simulink model "flightSimulation"  (R2018a)
settings: Solver=FixedStepAuto  StartTime=0  StopTime=end_time  FixedStep=0.005  RelTol=1e-3  EnableMultiTasking=on
values from neighbouring files (symbols this model uses):
  initPosLLA = [37.6287386167 -122.393391133 100]    [cmdh.mat]    (also in cmdyaw.mat)
  mass = 1.53    [cmdh.mat]    (also in cmdyaw.mat)
  Ts = 0.01    [cmdh.mat]    (also in cmdyaw.mat)
undefined symbols (not defined in the file or in its folder): B, Earth, ft, m, p_limits, s, sigbuilder_block, sw_turb, umax, umin, Vehicle, WGS84
libraries: simulink x23, aerolibactuator x15, dspswit3 x12, dspsrcs4 x10, dsparch4 x7, aerolibconvert2 x4, aerolibanimutils x2, qcatlib x2, aerolibfltsims x2, aerolibutil x2, shared6dof x1, aerolibtransform2 x1
(part 2 of 4)

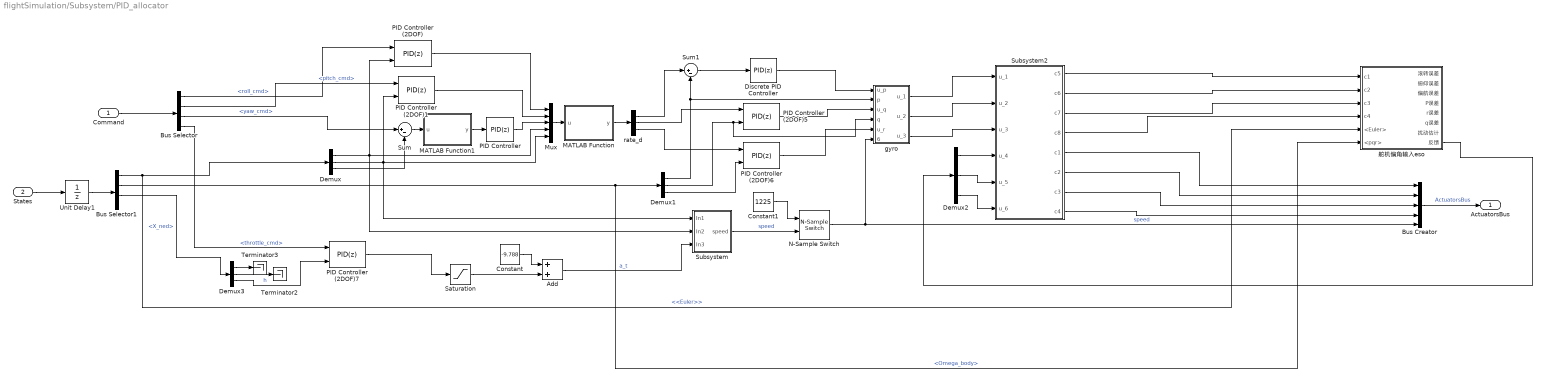
== system flightSimulation/Subsystem/PID_allocator ==
  Command : Inport
  States : Inport  Port=2  OutDataTypeStr=Bus: StatesBus
  Add : Sum
  Bus Creator : BusCreator  Inputs=5  OutDataTypeStr=Bus: ActuatorsBus
  Bus Selector : BusSelector  OutputSignals=roll_cmd,pitch_cmd,yaw_cmd,throttle_cmd
  Bus Selector1 : BusSelector  OutputSignals=<Euler>,Omega_body,X_ned,V_ned
  Constant : Constant  Value=-9.788
  Constant1 : Constant  Value=1225
  Demux{,1..3} (4 alike) : Demux  Outputs=3
  Discrete PID Controller : simulink/Continuous/PID Controller  Controller=PID  TimeDomain=Discrete-time  SampleTime=-1  IntegratorMethod=Forward Euler  FilterMethod=Forward Euler  Form=Parallel  UseFilter=on  ControllerParametersSource=internal  P=0.4  I=0.32  D=0  N=100  InitialConditionSource=internal  InitialConditionForIntegrator=0  InitialConditionForFilter=0  ExternalReset=none  LimitOutput=off  UpperSaturationLimit=inf  LowerSaturationLimit=-inf  LinearizeAsGain=off  AntiWindupMode=none  Kb=1  TrackingMode=off  Kt=1  PParamMin=[]  PParamMax=[]  IParamMin=[]  IParamMax=[]  DParamMin=[]  DParamMax=[]  NParamMin=[]  NParamMax=[]  KbParamMin=[]  KbParamMax=[]  KtParamMin=[]  KtParamMax=[]  POutMin=[]  POutMax=[]  IOutMin=[]  IOutMax=[]  DOutMin=[]  DOutMax=[]  NOutMin=[]  NOutMax=[]  KbOutMin=[]  KbOutMax=[]  KtOutMin=[]  KtOutMax=[]  IntegratorOutMin=[]  IntegratorOutMax=[]  FilterOutMin=[]  FilterOutMax=[]  SumOutMin=[]  SumOutMax=[]  SumI1OutMin=[]  SumI1OutMax=[]  SumI2OutMin=[]  SumI2OutMax=[]  SumI3OutMin=[]  SumI3OutMax=[]  SumDOutMin=[]  SumDOutMax=[]  SaturationOutMin=[]  SaturationOutMax=[]  IntegratorContinuousStateAttributes=''  IntegratorStateMustResolveToSignalObject=off  IntegratorRTWStateStorageClass=Auto  FilterContinuousStateAttributes=''  FilterStateMustResolveToSignalObject=off  FilterRTWStateStorageClass=Auto  DifferentiatorICPrevScaledInput=0  DifferentiatorOutMin=[]  DifferentiatorOutMax=[]  FilterDiffOutCoefMin=[]  FilterDiffOutCoefMax=[]  SumDenOutMin=[]  SumDenOutMax=[]  SumNumOutMin=[]  SumNumOutMax=[]  ReciprocalOutMin=[]  ReciprocalOutMax=[]  DivideOutMin=[]  DivideOutMax=[]  TunerSelectOption=Transfer Function Based (PID Tuner App)
  MATLAB Function : MATLAB Function  TreatAsAtomicUnit=on
  MATLAB Function1 : MATLAB Function  TreatAsAtomicUnit=on
  Mux : Mux  Inputs=5
  N-Sample Switch : dspswit3/N-Sample Switch  N=3  reset=off  TriggerType=Rising edge  Ts=0.01
      settings: SourceProductName=DSP System Toolbox  SourceProductBaseCode=DS
  PID Controller : simulink/Continuous/PID Controller  Controller=PID  TimeDomain=Discrete-time  SampleTime=-1  IntegratorMethod=Forward Euler  FilterMethod=Forward Euler  Form=Parallel  UseFilter=on  ControllerParametersSource=internal  P=3  I=0.2  D=0  N=100  InitialConditionSource=internal  InitialConditionForIntegrator=0  InitialConditionForFilter=0  ExternalReset=none  LimitOutput=off  UpperSaturationLimit=1*pi  LowerSaturationLimit=-1*pi  LinearizeAsGain=on  AntiWindupMode=none  Kb=1  TrackingMode=off  Kt=1  PParamMin=[]  PParamMax=[]  IParamMin=[]  IParamMax=[]  DParamMin=[]  DParamMax=[]  NParamMin=[]  NParamMax=[]  KbParamMin=[]  KbParamMax=[]  KtParamMin=[]  KtParamMax=[]  POutMin=[]  POutMax=[]  IOutMin=[]  IOutMax=[]  DOutMin=[]  DOutMax=[]  NOutMin=[]  NOutMax=[]  KbOutMin=[]  KbOutMax=[]  KtOutMin=[]  KtOutMax=[]  IntegratorOutMin=[]  IntegratorOutMax=[]  FilterOutMin=[]  FilterOutMax=[]  SumOutMin=[]  SumOutMax=[]  SumI1OutMin=[]  SumI1OutMax=[]  SumI2OutMin=[]  SumI2OutMax=[]  SumI3OutMin=[]  SumI3OutMax=[]  SumDOutMin=[]  SumDOutMax=[]  SaturationOutMin=[]  SaturationOutMax=[]  IntegratorContinuousStateAttributes=''  IntegratorStateMustResolveToSignalObject=off  IntegratorRTWStateStorageClass=Auto  FilterContinuousStateAttributes=''  FilterStateMustResolveToSignalObject=off  FilterRTWStateStorageClass=Auto  DifferentiatorICPrevScaledInput=0  DifferentiatorOutMin=[]  DifferentiatorOutMax=[]  FilterDiffOutCoefMin=[]  FilterDiffOutCoefMax=[]  SumDenOutMin=[]  SumDenOutMax=[]  SumNumOutMin=[]  SumNumOutMax=[]  ReciprocalOutMin=[]  ReciprocalOutMax=[]  DivideOutMin=[]  DivideOutMax=[]  TunerSelectOption=Transfer Function Based (PID Tuner App)
  PID Controller (2DOF) : simulink/Continuous/PID Controller (2DOF)  Controller=PID  TimeDomain=Discrete-time  SampleTime=-1  IntegratorMethod=Forward Euler  FilterMethod=Forward Euler  Form=Parallel  UseFilter=on  ControllerParametersSource=internal  P=4  I=0  D=0  N=100  b=1  c=1  InitialConditionSource=internal  InitialConditionForIntegrator=0  InitialConditionForFilter=0  ExternalReset=none  LimitOutput=off  UpperSaturationLimit=1*pi  LowerSaturationLimit=-1*pi  LinearizeAsGain=on  AntiWindupMode=none  Kb=1  TrackingMode=off  Kt=1  PParamMin=[]  PParamMax=[]  IParamMin=[]  IParamMax=[]  DParamMin=[]  DParamMax=[]  NParamMin=[]  NParamMax=[]  bParamMin=[]  bParamMax=[]  cParamMin=[]  cParamMax=[]  KbParamMin=[]  KbParamMax=[]  KtParamMin=[]  KtParamMax=[]  POutMin=[]  POutMax=[]  IOutMin=[]  IOutMax=[]  DOutMin=[]  DOutMax=[]  NOutMin=[]  NOutMax=[]  bOutMin=[]  bOutMax=[]  cOutMin=[]  cOutMax=[]  KbOutMin=[]  KbOutMax=[]  KtOutMin=[]  KtOutMax=[]  IntegratorOutMin=[]  IntegratorOutMax=[]  FilterOutMin=[]  FilterOutMax=[]  SumOutMin=[]  SumOutMax=[]  Sum1OutMin=[]  Sum1OutMax=[]  Sum2OutMin=[]  Sum2OutMax=[]  Sum3OutMin=[]  Sum3OutMax=[]  SumI1OutMin=[]  SumI1OutMax=[]  SumI2OutMin=[]  SumI2OutMax=[]  SumI3OutMin=[]  SumI3OutMax=[]  SumDOutMin=[]  SumDOutMax=[]  SaturationOutMin=[]  SaturationOutMax=[]  IntegratorContinuousStateAttributes=''  IntegratorStateMustResolveToSignalObject=off  IntegratorRTWStateStorageClass=Auto  FilterContinuousStateAttributes=''  FilterStateMustResolveToSignalObject=off  FilterRTWStateStorageClass=Auto  DifferentiatorICPrevScaledInput=0  DifferentiatorOutMin=[]  DifferentiatorOutMax=[]  FilterDiffOutCoefMin=[]  FilterDiffOutCoefMax=[]  SumDenOutMin=[]  SumDenOutMax=[]  SumNumOutMin=[]  SumNumOutMax=[]  ReciprocalOutMin=[]  ReciprocalOutMax=[]  DivideOutMin=[]  DivideOutMax=[]  TunerSelectOption=Transfer Function Based (PID Tuner App)
  PID Controller (2DOF)1 : simulink/Continuous/PID Controller (2DOF)  Controller=PID  TimeDomain=Discrete-time  SampleTime=-1  IntegratorMethod=Forward Euler  FilterMethod=Forward Euler  Form=Parallel  UseFilter=on  ControllerParametersSource=internal  P=4  I=0  D=0  N=100  b=1  c=1  InitialConditionSource=internal  InitialConditionForIntegrator=0  InitialConditionForFilter=0  ExternalReset=none  LimitOutput=off  UpperSaturationLimit=1*pi  LowerSaturationLimit=-1*pi  LinearizeAsGain=on  AntiWindupMode=none  Kb=1  TrackingMode=off  Kt=1  PParamMin=[]  PParamMax=[]  IParamMin=[]  IParamMax=[]  DParamMin=[]  DParamMax=[]  NParamMin=[]  NParamMax=[]  bParamMin=[]  bParamMax=[]  cParamMin=[]  cParamMax=[]  KbParamMin=[]  KbParamMax=[]  KtParamMin=[]  KtParamMax=[]  POutMin=[]  POutMax=[]  IOutMin=[]  IOutMax=[]  DOutMin=[]  DOutMax=[]  NOutMin=[]  NOutMax=[]  bOutMin=[]  bOutMax=[]  cOutMin=[]  cOutMax=[]  KbOutMin=[]  KbOutMax=[]  KtOutMin=[]  KtOutMax=[]  IntegratorOutMin=[]  IntegratorOutMax=[]  FilterOutMin=[]  FilterOutMax=[]  SumOutMin=[]  SumOutMax=[]  Sum1OutMin=[]  Sum1OutMax=[]  Sum2OutMin=[]  Sum2OutMax=[]  Sum3OutMin=[]  Sum3OutMax=[]  SumI1OutMin=[]  SumI1OutMax=[]  SumI2OutMin=[]  SumI2OutMax=[]  SumI3OutMin=[]  SumI3OutMax=[]  SumDOutMin=[]  SumDOutMax=[]  SaturationOutMin=[]  SaturationOutMax=[]  IntegratorContinuousStateAttributes=''  IntegratorStateMustResolveToSignalObject=off  IntegratorRTWStateStorageClass=Auto  FilterContinuousStateAttributes=''  FilterStateMustResolveToSignalObject=off  FilterRTWStateStorageClass=Auto  DifferentiatorICPrevScaledInput=0  DifferentiatorOutMin=[]  DifferentiatorOutMax=[]  FilterDiffOutCoefMin=[]  FilterDiffOutCoefMax=[]  SumDenOutMin=[]  SumDenOutMax=[]  SumNumOutMin=[]  SumNumOutMax=[]  ReciprocalOutMin=[]  ReciprocalOutMax=[]  DivideOutMin=[]  DivideOutMax=[]  TunerSelectOption=Transfer Function Based (PID Tuner App)
  PID Controller (2DOF)5 : simulink/Continuous/PID Controller (2DOF)  Controller=PID  TimeDomain=Discrete-time  SampleTime=-1  IntegratorMethod=Forward Euler  FilterMethod=Forward Euler  Form=Parallel  UseFilter=on  ControllerParametersSource=internal  P=0.4  I=0.32  D=0  N=100  b=1  c=1  InitialConditionSource=internal  InitialConditionForIntegrator=0  InitialConditionForFilter=0  ExternalReset=none  LimitOutput=off  UpperSaturationLimit=inf  LowerSaturationLimit=-inf  LinearizeAsGain=on  AntiWindupMode=none  Kb=1  TrackingMode=off  Kt=1  PParamMin=[]  PParamMax=[]  IParamMin=[]  IParamMax=[]  DParamMin=[]  DParamMax=[]  NParamMin=[]  NParamMax=[]  bParamMin=[]  bParamMax=[]  cParamMin=[]  cParamMax=[]  KbParamMin=[]  KbParamMax=[]  KtParamMin=[]  KtParamMax=[]  POutMin=[]  POutMax=[]  IOutMin=[]  IOutMax=[]  DOutMin=[]  DOutMax=[]  NOutMin=[]  NOutMax=[]  bOutMin=[]  bOutMax=[]  cOutMin=[]  cOutMax=[]  KbOutMin=[]  KbOutMax=[]  KtOutMin=[]  KtOutMax=[]  IntegratorOutMin=[]  IntegratorOutMax=[]  FilterOutMin=[]  FilterOutMax=[]  SumOutMin=[]  SumOutMax=[]  Sum1OutMin=[]  Sum1OutMax=[]  Sum2OutMin=[]  Sum2OutMax=[]  Sum3OutMin=[]  Sum3OutMax=[]  SumI1OutMin=[]  SumI1OutMax=[]  SumI2OutMin=[]  SumI2OutMax=[]  SumI3OutMin=[]  SumI3OutMax=[]  SumDOutMin=[]  SumDOutMax=[]  SaturationOutMin=[]  SaturationOutMax=[]  IntegratorContinuousStateAttributes=''  IntegratorStateMustResolveToSignalObject=off  IntegratorRTWStateStorageClass=Auto  FilterContinuousStateAttributes=''  FilterStateMustResolveToSignalObject=off  FilterRTWStateStorageClass=Auto  DifferentiatorICPrevScaledInput=0  DifferentiatorOutMin=[]  DifferentiatorOutMax=[]  FilterDiffOutCoefMin=[]  FilterDiffOutCoefMax=[]  SumDenOutMin=[]  SumDenOutMax=[]  SumNumOutMin=[]  SumNumOutMax=[]  ReciprocalOutMin=[]  ReciprocalOutMax=[]  DivideOutMin=[]  DivideOutMax=[]  TunerSelectOption=Transfer Function Based (PID Tuner App)
  PID Controller (2DOF)6 : simulink/Continuous/PID Controller (2DOF)  Controller=PID  TimeDomain=Discrete-time  SampleTime=-1  IntegratorMethod=Forward Euler  FilterMethod=Forward Euler  Form=Parallel  UseFilter=on  ControllerParametersSource=internal  P=0.25  I=0.5  D=0  N=100  b=1  c=1  InitialConditionSource=internal  InitialConditionForIntegrator=0  InitialConditionForFilter=0  ExternalReset=none  LimitOutput=off  UpperSaturationLimit=inf  LowerSaturationLimit=-inf  LinearizeAsGain=on  AntiWindupMode=none  Kb=1  TrackingMode=off  Kt=1  PParamMin=[]  PParamMax=[]  IParamMin=[]  IParamMax=[]  DParamMin=[]  DParamMax=[]  NParamMin=[]  NParamMax=[]  bParamMin=[]  bParamMax=[]  cParamMin=[]  cParamMax=[]  KbParamMin=[]  KbParamMax=[]  KtParamMin=[]  KtParamMax=[]  POutMin=[]  POutMax=[]  IOutMin=[]  IOutMax=[]  DOutMin=[]  DOutMax=[]  NOutMin=[]  NOutMax=[]  bOutMin=[]  bOutMax=[]  cOutMin=[]  cOutMax=[]  KbOutMin=[]  KbOutMax=[]  KtOutMin=[]  KtOutMax=[]  IntegratorOutMin=[]  IntegratorOutMax=[]  FilterOutMin=[]  FilterOutMax=[]  SumOutMin=[]  SumOutMax=[]  Sum1OutMin=[]  Sum1OutMax=[]  Sum2OutMin=[]  Sum2OutMax=[]  Sum3OutMin=[]  Sum3OutMax=[]  SumI1OutMin=[]  SumI1OutMax=[]  SumI2OutMin=[]  SumI2OutMax=[]  SumI3OutMin=[]  SumI3OutMax=[]  SumDOutMin=[]  SumDOutMax=[]  SaturationOutMin=[]  SaturationOutMax=[]  IntegratorContinuousStateAttributes=''  IntegratorStateMustResolveToSignalObject=off  IntegratorRTWStateStorageClass=Auto  FilterContinuousStateAttributes=''  FilterStateMustResolveToSignalObject=off  FilterRTWStateStorageClass=Auto  DifferentiatorICPrevScaledInput=0  DifferentiatorOutMin=[]  DifferentiatorOutMax=[]  FilterDiffOutCoefMin=[]  FilterDiffOutCoefMax=[]  SumDenOutMin=[]  SumDenOutMax=[]  SumNumOutMin=[]  SumNumOutMax=[]  ReciprocalOutMin=[]  ReciprocalOutMax=[]  DivideOutMin=[]  DivideOutMax=[]  TunerSelectOption=Transfer Function Based (PID Tuner App)
  PID Controller (2DOF)7 : simulink/Continuous/PID Controller (2DOF)  Controller=PID  TimeDomain=Discrete-time  SampleTime=-1  IntegratorMethod=Forward Euler  FilterMethod=Forward Euler  Form=Parallel  UseFilter=on  ControllerParametersSource=internal  P=2.1  I=0.2  D=2.1  N=100  b=1  c=1  InitialConditionSource=internal  InitialConditionForIntegrator=0  InitialConditionForFilter=0  ExternalReset=none  LimitOutput=off  UpperSaturationLimit=inf  LowerSaturationLimit=-inf  LinearizeAsGain=on  AntiWindupMode=none  Kb=1  TrackingMode=off  Kt=1  PParamMin=[]  PParamMax=[]  IParamMin=[]  IParamMax=[]  DParamMin=[]  DParamMax=[]  NParamMin=[]  NParamMax=[]  bParamMin=[]  bParamMax=[]  cParamMin=[]  cParamMax=[]  KbParamMin=[]  KbParamMax=[]  KtParamMin=[]  KtParamMax=[]  POutMin=[]  POutMax=[]  IOutMin=[]  IOutMax=[]  DOutMin=[]  DOutMax=[]  NOutMin=[]  NOutMax=[]  bOutMin=[]  bOutMax=[]  cOutMin=[]  cOutMax=[]  KbOutMin=[]  KbOutMax=[]  KtOutMin=[]  KtOutMax=[]  IntegratorOutMin=[]  IntegratorOutMax=[]  FilterOutMin=[]  FilterOutMax=[]  SumOutMin=[]  SumOutMax=[]  Sum1OutMin=[]  Sum1OutMax=[]  Sum2OutMin=[]  Sum2OutMax=[]  Sum3OutMin=[]  Sum3OutMax=[]  SumI1OutMin=[]  SumI1OutMax=[]  SumI2OutMin=[]  SumI2OutMax=[]  SumI3OutMin=[]  SumI3OutMax=[]  SumDOutMin=[]  SumDOutMax=[]  SaturationOutMin=[]  SaturationOutMax=[]  IntegratorContinuousStateAttributes=''  IntegratorStateMustResolveToSignalObject=off  IntegratorRTWStateStorageClass=Auto  FilterContinuousStateAttributes=''  FilterStateMustResolveToSignalObject=off  FilterRTWStateStorageClass=Auto  DifferentiatorICPrevScaledInput=0  DifferentiatorOutMin=[]  DifferentiatorOutMax=[]  FilterDiffOutCoefMin=[]  FilterDiffOutCoefMax=[]  SumDenOutMin=[]  SumDenOutMax=[]  SumNumOutMin=[]  SumNumOutMax=[]  ReciprocalOutMin=[]  ReciprocalOutMax=[]  DivideOutMin=[]  DivideOutMax=[]  TunerSelectOption=Transfer Function Based (PID Tuner App)
  Saturation : Saturate  UpperLimit=9.788  LowerLimit=-9.788
  Subsystem : Subsystem
  Subsystem2 : Subsystem
  Sum : Sum  Inputs=|+-
  Sum1 : Sum  Inputs=|+-
  Terminator2 : Terminator
  Terminator3 : Terminator
  Unit Delay1 : UnitDelay  SampleTime=-1
  gyro : Subsystem
  rate_d : Demux  Outputs=3
  舵机偏角输入eso : Subsystem
  ActuatorsBus : Outport  OutDataTypeStr=Bus: ActuatorsBus
  wires:
  PID Controller/1 -> Mux/3
  Bus Selector/3 -> Sum/1  "<yaw_cmd>"
  Demux/3 -> Sum/2
  PID Controller (2DOF)7/1 -> Saturation/1
  Bus Selector/2 -> PID Controller (2DOF)1/1  "<pitch_cmd>"
  Bus Selector1/2 -> Demux1/1, 舵机偏角输入eso/6(<pqr>)  "<Omega_body>"
  Sum/1 -> MATLAB Function1/1(u)
  PID Controller (2DOF)/1 -> Mux/1
  Demux3/2 -> Terminator2/1
  Demux/2 -> PID Controller (2DOF)1/2, Mux/5, Subsystem/1(In1)
  Demux1/2 -> gyro/4(q), PID Controller (2DOF)5/2
  rate_d/3 -> PID Controller (2DOF)6/1
  PID Controller (2DOF)1/1 -> Mux/2
  Demux1/3 -> PID Controller (2DOF)6/2
  MATLAB Function1/1(y) -> PID Controller/1
  Demux3/1 -> Terminator3/1
  rate_d/2 -> PID Controller (2DOF)5/1
  Bus Selector/4 -> PID Controller (2DOF)7/1  "<throttle_cmd>"
  rate_d/1 -> Sum1/1
  Mux/1 -> MATLAB Function/1(u)
  Command/1 -> Bus Selector/1
  Bus Creator/1 -> ActuatorsBus/1  "ActuatorsBus"
  Constant1/1 -> N-Sample Switch/1
  Subsystem/1(speed) -> N-Sample Switch/2  "speed"
  N-Sample Switch/1 -> gyro/6(speed), Bus Creator/5  "speed"
  Demux3/3 -> PID Controller (2DOF)7/2  "h"
  MATLAB Function/1(y) -> rate_d/1
  States/1 -> Unit Delay1/1
  Unit Delay1/1 -> Bus Selector1/1
  Add/1 -> Subsystem/3(In3)  "a_t"
  Constant/1 -> Add/1
  Sum1/1 -> Discrete PID Controller/1
  Bus Selector/1 -> PID Controller (2DOF)/1  "<roll_cmd>"
  Saturation/1 -> Add/2
  Demux/1 -> PID Controller (2DOF)/2, Subsystem/2(In2), Mux/4
  Demux1/1 -> gyro/2(p), Sum1/2
  Subsystem2/5(c1) -> Bus Creator/1
  Subsystem2/7(c3) -> Bus Creator/3
  Subsystem2/6(c2) -> Bus Creator/2
  Bus Selector1/3 -> Demux3/1  "<X_ned>"
  Subsystem2/8(c4) -> Bus Creator/4
  Bus Selector1/1 -> Demux/1, 舵机偏角输入eso/5(<Euler>)  "<<Euler>>"
  Discrete PID Controller/1 -> gyro/1(u_p)
  PID Controller (2DOF)5/1 -> gyro/3(u_q)
  PID Controller (2DOF)6/1 -> gyro/5(u_r)
  Demux2/1 -> Subsystem2/4(u_4)
  Demux2/2 -> Subsystem2/5(u_5)
  Demux2/3 -> Subsystem2/6(u_6)
  Subsystem2/1(c5) -> 舵机偏角输入eso/1(c1)
  Subsystem2/2(c6) -> 舵机偏角输入eso/2(c2)
  Subsystem2/3(c7) -> 舵机偏角输入eso/3(c3)
  Subsystem2/4(c8) -> 舵机偏角输入eso/4(c4)
  gyro/1(u_1) -> Subsystem2/1(u_1)
  gyro/2(u_2) -> Subsystem2/2(u_2)
  gyro/3(u_3) -> Subsystem2/3(u_3)
  舵机偏角输入eso/8(反馈) -> Demux2/1

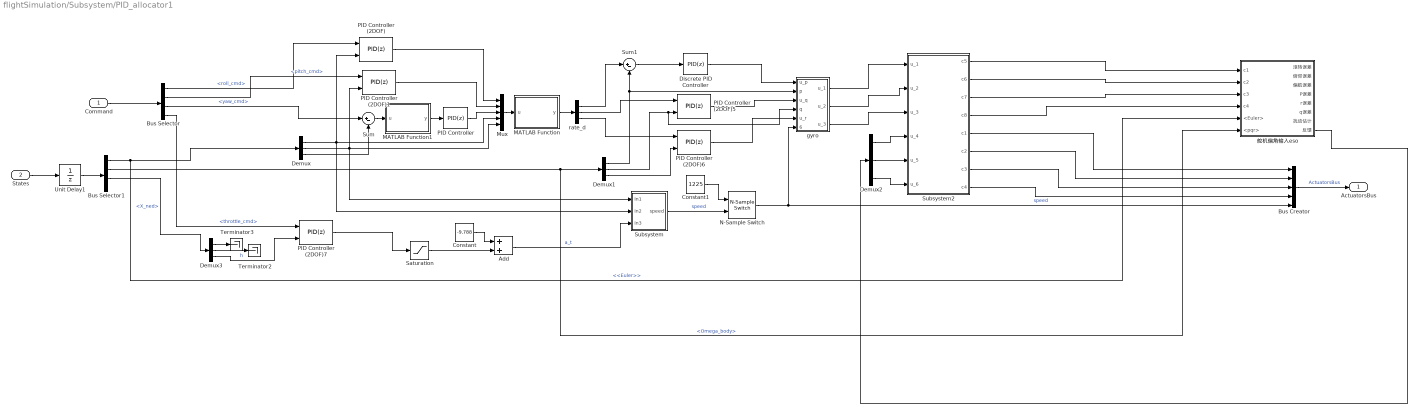
== system flightSimulation/Subsystem/PID_allocator1 ==
  Command : Inport
  States : Inport  Port=2  OutDataTypeStr=Bus: StatesBus
  Add : Sum
  Bus Creator : BusCreator  Inputs=5  OutDataTypeStr=Bus: ActuatorsBus
  Bus Selector : BusSelector  OutputSignals=roll_cmd,pitch_cmd,yaw_cmd,throttle_cmd
  Bus Selector1 : BusSelector  OutputSignals=<Euler>,Omega_body,X_ned,V_ned
  Constant : Constant  Value=-9.788
  Constant1 : Constant  Value=1225
  Demux{,1..3} (4 alike) : Demux  Outputs=3
  Discrete PID Controller : simulink/Continuous/PID Controller  Controller=PID  TimeDomain=Discrete-time  SampleTime=-1  IntegratorMethod=Forward Euler  FilterMethod=Forward Euler  Form=Parallel  UseFilter=on  ControllerParametersSource=internal  P=0.4  I=0.32  D=0  N=100  InitialConditionSource=internal  InitialConditionForIntegrator=0  InitialConditionForFilter=0  ExternalReset=none  LimitOutput=off  UpperSaturationLimit=inf  LowerSaturationLimit=-inf  LinearizeAsGain=off  AntiWindupMode=none  Kb=1  TrackingMode=off  Kt=1  PParamMin=[]  PParamMax=[]  IParamMin=[]  IParamMax=[]  DParamMin=[]  DParamMax=[]  NParamMin=[]  NParamMax=[]  KbParamMin=[]  KbParamMax=[]  KtParamMin=[]  KtParamMax=[]  POutMin=[]  POutMax=[]  IOutMin=[]  IOutMax=[]  DOutMin=[]  DOutMax=[]  NOutMin=[]  NOutMax=[]  KbOutMin=[]  KbOutMax=[]  KtOutMin=[]  KtOutMax=[]  IntegratorOutMin=[]  IntegratorOutMax=[]  FilterOutMin=[]  FilterOutMax=[]  SumOutMin=[]  SumOutMax=[]  SumI1OutMin=[]  SumI1OutMax=[]  SumI2OutMin=[]  SumI2OutMax=[]  SumI3OutMin=[]  SumI3OutMax=[]  SumDOutMin=[]  SumDOutMax=[]  SaturationOutMin=[]  SaturationOutMax=[]  IntegratorContinuousStateAttributes=''  IntegratorStateMustResolveToSignalObject=off  IntegratorRTWStateStorageClass=Auto  FilterContinuousStateAttributes=''  FilterStateMustResolveToSignalObject=off  FilterRTWStateStorageClass=Auto  DifferentiatorICPrevScaledInput=0  DifferentiatorOutMin=[]  DifferentiatorOutMax=[]  FilterDiffOutCoefMin=[]  FilterDiffOutCoefMax=[]  SumDenOutMin=[]  SumDenOutMax=[]  SumNumOutMin=[]  SumNumOutMax=[]  ReciprocalOutMin=[]  ReciprocalOutMax=[]  DivideOutMin=[]  DivideOutMax=[]  TunerSelectOption=Transfer Function Based (PID Tuner App)
  MATLAB Function : MATLAB Function  TreatAsAtomicUnit=on
  MATLAB Function1 : MATLAB Function  TreatAsAtomicUnit=on
  Mux : Mux  Inputs=5
  N-Sample Switch : dspswit3/N-Sample Switch  N=3  reset=off  TriggerType=Rising edge  Ts=0.01
      settings: SourceProductName=DSP System Toolbox  SourceProductBaseCode=DS
  PID Controller : simulink/Continuous/PID Controller  Controller=PID  TimeDomain=Discrete-time  SampleTime=-1  IntegratorMethod=Forward Euler  FilterMethod=Forward Euler  Form=Parallel  UseFilter=on  ControllerParametersSource=internal  P=3  I=0.2  D=0  N=100  InitialConditionSource=internal  InitialConditionForIntegrator=0  InitialConditionForFilter=0  ExternalReset=none  LimitOutput=off  UpperSaturationLimit=1*pi  LowerSaturationLimit=-1*pi  LinearizeAsGain=on  AntiWindupMode=none  Kb=1  TrackingMode=off  Kt=1  PParamMin=[]  PParamMax=[]  IParamMin=[]  IParamMax=[]  DParamMin=[]  DParamMax=[]  NParamMin=[]  NParamMax=[]  KbParamMin=[]  KbParamMax=[]  KtParamMin=[]  KtParamMax=[]  POutMin=[]  POutMax=[]  IOutMin=[]  IOutMax=[]  DOutMin=[]  DOutMax=[]  NOutMin=[]  NOutMax=[]  KbOutMin=[]  KbOutMax=[]  KtOutMin=[]  KtOutMax=[]  IntegratorOutMin=[]  IntegratorOutMax=[]  FilterOutMin=[]  FilterOutMax=[]  SumOutMin=[]  SumOutMax=[]  SumI1OutMin=[]  SumI1OutMax=[]  SumI2OutMin=[]  SumI2OutMax=[]  SumI3OutMin=[]  SumI3OutMax=[]  SumDOutMin=[]  SumDOutMax=[]  SaturationOutMin=[]  SaturationOutMax=[]  IntegratorContinuousStateAttributes=''  IntegratorStateMustResolveToSignalObject=off  IntegratorRTWStateStorageClass=Auto  FilterContinuousStateAttributes=''  FilterStateMustResolveToSignalObject=off  FilterRTWStateStorageClass=Auto  DifferentiatorICPrevScaledInput=0  DifferentiatorOutMin=[]  DifferentiatorOutMax=[]  FilterDiffOutCoefMin=[]  FilterDiffOutCoefMax=[]  SumDenOutMin=[]  SumDenOutMax=[]  SumNumOutMin=[]  SumNumOutMax=[]  ReciprocalOutMin=[]  ReciprocalOutMax=[]  DivideOutMin=[]  DivideOutMax=[]  TunerSelectOption=Transfer Function Based (PID Tuner App)
  PID Controller (2DOF) : simulink/Continuous/PID Controller (2DOF)  Controller=PID  TimeDomain=Discrete-time  SampleTime=-1  IntegratorMethod=Forward Euler  FilterMethod=Forward Euler  Form=Parallel  UseFilter=on  ControllerParametersSource=internal  P=4  I=0  D=0  N=100  b=1  c=1  InitialConditionSource=internal  InitialConditionForIntegrator=0  InitialConditionForFilter=0  ExternalReset=none  LimitOutput=off  UpperSaturationLimit=1*pi  LowerSaturationLimit=-1*pi  LinearizeAsGain=on  AntiWindupMode=none  Kb=1  TrackingMode=off  Kt=1  PParamMin=[]  PParamMax=[]  IParamMin=[]  IParamMax=[]  DParamMin=[]  DParamMax=[]  NParamMin=[]  NParamMax=[]  bParamMin=[]  bParamMax=[]  cParamMin=[]  cParamMax=[]  KbParamMin=[]  KbParamMax=[]  KtParamMin=[]  KtParamMax=[]  POutMin=[]  POutMax=[]  IOutMin=[]  IOutMax=[]  DOutMin=[]  DOutMax=[]  NOutMin=[]  NOutMax=[]  bOutMin=[]  bOutMax=[]  cOutMin=[]  cOutMax=[]  KbOutMin=[]  KbOutMax=[]  KtOutMin=[]  KtOutMax=[]  IntegratorOutMin=[]  IntegratorOutMax=[]  FilterOutMin=[]  FilterOutMax=[]  SumOutMin=[]  SumOutMax=[]  Sum1OutMin=[]  Sum1OutMax=[]  Sum2OutMin=[]  Sum2OutMax=[]  Sum3OutMin=[]  Sum3OutMax=[]  SumI1OutMin=[]  SumI1OutMax=[]  SumI2OutMin=[]  SumI2OutMax=[]  SumI3OutMin=[]  SumI3OutMax=[]  SumDOutMin=[]  SumDOutMax=[]  SaturationOutMin=[]  SaturationOutMax=[]  IntegratorContinuousStateAttributes=''  IntegratorStateMustResolveToSignalObject=off  IntegratorRTWStateStorageClass=Auto  FilterContinuousStateAttributes=''  FilterStateMustResolveToSignalObject=off  FilterRTWStateStorageClass=Auto  DifferentiatorICPrevScaledInput=0  DifferentiatorOutMin=[]  DifferentiatorOutMax=[]  FilterDiffOutCoefMin=[]  FilterDiffOutCoefMax=[]  SumDenOutMin=[]  SumDenOutMax=[]  SumNumOutMin=[]  SumNumOutMax=[]  ReciprocalOutMin=[]  ReciprocalOutMax=[]  DivideOutMin=[]  DivideOutMax=[]  TunerSelectOption=Transfer Function Based (PID Tuner App)
  PID Controller (2DOF)1 : simulink/Continuous/PID Controller (2DOF)  Controller=PID  TimeDomain=Discrete-time  SampleTime=-1  IntegratorMethod=Forward Euler  FilterMethod=Forward Euler  Form=Parallel  UseFilter=on  ControllerParametersSource=internal  P=4  I=0  D=0  N=100  b=1  c=1  InitialConditionSource=internal  InitialConditionForIntegrator=0  InitialConditionForFilter=0  ExternalReset=none  LimitOutput=off  UpperSaturationLimit=1*pi  LowerSaturationLimit=-1*pi  LinearizeAsGain=on  AntiWindupMode=none  Kb=1  TrackingMode=off  Kt=1  PParamMin=[]  PParamMax=[]  IParamMin=[]  IParamMax=[]  DParamMin=[]  DParamMax=[]  NParamMin=[]  NParamMax=[]  bParamMin=[]  bParamMax=[]  cParamMin=[]  cParamMax=[]  KbParamMin=[]  KbParamMax=[]  KtParamMin=[]  KtParamMax=[]  POutMin=[]  POutMax=[]  IOutMin=[]  IOutMax=[]  DOutMin=[]  DOutMax=[]  NOutMin=[]  NOutMax=[]  bOutMin=[]  bOutMax=[]  cOutMin=[]  cOutMax=[]  KbOutMin=[]  KbOutMax=[]  KtOutMin=[]  KtOutMax=[]  IntegratorOutMin=[]  IntegratorOutMax=[]  FilterOutMin=[]  FilterOutMax=[]  SumOutMin=[]  SumOutMax=[]  Sum1OutMin=[]  Sum1OutMax=[]  Sum2OutMin=[]  Sum2OutMax=[]  Sum3OutMin=[]  Sum3OutMax=[]  SumI1OutMin=[]  SumI1OutMax=[]  SumI2OutMin=[]  SumI2OutMax=[]  SumI3OutMin=[]  SumI3OutMax=[]  SumDOutMin=[]  SumDOutMax=[]  SaturationOutMin=[]  SaturationOutMax=[]  IntegratorContinuousStateAttributes=''  IntegratorStateMustResolveToSignalObject=off  IntegratorRTWStateStorageClass=Auto  FilterContinuousStateAttributes=''  FilterStateMustResolveToSignalObject=off  FilterRTWStateStorageClass=Auto  DifferentiatorICPrevScaledInput=0  DifferentiatorOutMin=[]  DifferentiatorOutMax=[]  FilterDiffOutCoefMin=[]  FilterDiffOutCoefMax=[]  SumDenOutMin=[]  SumDenOutMax=[]  SumNumOutMin=[]  SumNumOutMax=[]  ReciprocalOutMin=[]  ReciprocalOutMax=[]  DivideOutMin=[]  DivideOutMax=[]  TunerSelectOption=Transfer Function Based (PID Tuner App)
  PID Controller (2DOF)5 : simulink/Continuous/PID Controller (2DOF)  Controller=PID  TimeDomain=Discrete-time  SampleTime=-1  IntegratorMethod=Forward Euler  FilterMethod=Forward Euler  Form=Parallel  UseFilter=on  ControllerParametersSource=internal  P=0.4  I=0.32  D=0  N=100  b=1  c=1  InitialConditionSource=internal  InitialConditionForIntegrator=0  InitialConditionForFilter=0  ExternalReset=none  LimitOutput=off  UpperSaturationLimit=inf  LowerSaturationLimit=-inf  LinearizeAsGain=on  AntiWindupMode=none  Kb=1  TrackingMode=off  Kt=1  PParamMin=[]  PParamMax=[]  IParamMin=[]  IParamMax=[]  DParamMin=[]  DParamMax=[]  NParamMin=[]  NParamMax=[]  bParamMin=[]  bParamMax=[]  cParamMin=[]  cParamMax=[]  KbParamMin=[]  KbParamMax=[]  KtParamMin=[]  KtParamMax=[]  POutMin=[]  POutMax=[]  IOutMin=[]  IOutMax=[]  DOutMin=[]  DOutMax=[]  NOutMin=[]  NOutMax=[]  bOutMin=[]  bOutMax=[]  cOutMin=[]  cOutMax=[]  KbOutMin=[]  KbOutMax=[]  KtOutMin=[]  KtOutMax=[]  IntegratorOutMin=[]  IntegratorOutMax=[]  FilterOutMin=[]  FilterOutMax=[]  SumOutMin=[]  SumOutMax=[]  Sum1OutMin=[]  Sum1OutMax=[]  Sum2OutMin=[]  Sum2OutMax=[]  Sum3OutMin=[]  Sum3OutMax=[]  SumI1OutMin=[]  SumI1OutMax=[]  SumI2OutMin=[]  SumI2OutMax=[]  SumI3OutMin=[]  SumI3OutMax=[]  SumDOutMin=[]  SumDOutMax=[]  SaturationOutMin=[]  SaturationOutMax=[]  IntegratorContinuousStateAttributes=''  IntegratorStateMustResolveToSignalObject=off  IntegratorRTWStateStorageClass=Auto  FilterContinuousStateAttributes=''  FilterStateMustResolveToSignalObject=off  FilterRTWStateStorageClass=Auto  DifferentiatorICPrevScaledInput=0  DifferentiatorOutMin=[]  DifferentiatorOutMax=[]  FilterDiffOutCoefMin=[]  FilterDiffOutCoefMax=[]  SumDenOutMin=[]  SumDenOutMax=[]  SumNumOutMin=[]  SumNumOutMax=[]  ReciprocalOutMin=[]  ReciprocalOutMax=[]  DivideOutMin=[]  DivideOutMax=[]  TunerSelectOption=Transfer Function Based (PID Tuner App)
  PID Controller (2DOF)6 : simulink/Continuous/PID Controller (2DOF)  Controller=PID  TimeDomain=Discrete-time  SampleTime=-1  IntegratorMethod=Forward Euler  FilterMethod=Forward Euler  Form=Parallel  UseFilter=on  ControllerParametersSource=internal  P=0.25  I=0.5  D=0  N=100  b=1  c=1  InitialConditionSource=internal  InitialConditionForIntegrator=0  InitialConditionForFilter=0  ExternalReset=none  LimitOutput=off  UpperSaturationLimit=inf  LowerSaturationLimit=-inf  LinearizeAsGain=on  AntiWindupMode=none  Kb=1  TrackingMode=off  Kt=1  PParamMin=[]  PParamMax=[]  IParamMin=[]  IParamMax=[]  DParamMin=[]  DParamMax=[]  NParamMin=[]  NParamMax=[]  bParamMin=[]  bParamMax=[]  cParamMin=[]  cParamMax=[]  KbParamMin=[]  KbParamMax=[]  KtParamMin=[]  KtParamMax=[]  POutMin=[]  POutMax=[]  IOutMin=[]  IOutMax=[]  DOutMin=[]  DOutMax=[]  NOutMin=[]  NOutMax=[]  bOutMin=[]  bOutMax=[]  cOutMin=[]  cOutMax=[]  KbOutMin=[]  KbOutMax=[]  KtOutMin=[]  KtOutMax=[]  IntegratorOutMin=[]  IntegratorOutMax=[]  FilterOutMin=[]  FilterOutMax=[]  SumOutMin=[]  SumOutMax=[]  Sum1OutMin=[]  Sum1OutMax=[]  Sum2OutMin=[]  Sum2OutMax=[]  Sum3OutMin=[]  Sum3OutMax=[]  SumI1OutMin=[]  SumI1OutMax=[]  SumI2OutMin=[]  SumI2OutMax=[]  SumI3OutMin=[]  SumI3OutMax=[]  SumDOutMin=[]  SumDOutMax=[]  SaturationOutMin=[]  SaturationOutMax=[]  IntegratorContinuousStateAttributes=''  IntegratorStateMustResolveToSignalObject=off  IntegratorRTWStateStorageClass=Auto  FilterContinuousStateAttributes=''  FilterStateMustResolveToSignalObject=off  FilterRTWStateStorageClass=Auto  DifferentiatorICPrevScaledInput=0  DifferentiatorOutMin=[]  DifferentiatorOutMax=[]  FilterDiffOutCoefMin=[]  FilterDiffOutCoefMax=[]  SumDenOutMin=[]  SumDenOutMax=[]  SumNumOutMin=[]  SumNumOutMax=[]  ReciprocalOutMin=[]  ReciprocalOutMax=[]  DivideOutMin=[]  DivideOutMax=[]  TunerSelectOption=Transfer Function Based (PID Tuner App)
  PID Controller (2DOF)7 : simulink/Continuous/PID Controller (2DOF)  Controller=PID  TimeDomain=Discrete-time  SampleTime=-1  IntegratorMethod=Forward Euler  FilterMethod=Forward Euler  Form=Parallel  UseFilter=on  ControllerParametersSource=internal  P=2.1  I=0.2  D=2.1  N=100  b=1  c=1  InitialConditionSource=internal  InitialConditionForIntegrator=0  InitialConditionForFilter=0  ExternalReset=none  LimitOutput=off  UpperSaturationLimit=inf  LowerSaturationLimit=-inf  LinearizeAsGain=on  AntiWindupMode=none  Kb=1  TrackingMode=off  Kt=1  PParamMin=[]  PParamMax=[]  IParamMin=[]  IParamMax=[]  DParamMin=[]  DParamMax=[]  NParamMin=[]  NParamMax=[]  bParamMin=[]  bParamMax=[]  cParamMin=[]  cParamMax=[]  KbParamMin=[]  KbParamMax=[]  KtParamMin=[]  KtParamMax=[]  POutMin=[]  POutMax=[]  IOutMin=[]  IOutMax=[]  DOutMin=[]  DOutMax=[]  NOutMin=[]  NOutMax=[]  bOutMin=[]  bOutMax=[]  cOutMin=[]  cOutMax=[]  KbOutMin=[]  KbOutMax=[]  KtOutMin=[]  KtOutMax=[]  IntegratorOutMin=[]  IntegratorOutMax=[]  FilterOutMin=[]  FilterOutMax=[]  SumOutMin=[]  SumOutMax=[]  Sum1OutMin=[]  Sum1OutMax=[]  Sum2OutMin=[]  Sum2OutMax=[]  Sum3OutMin=[]  Sum3OutMax=[]  SumI1OutMin=[]  SumI1OutMax=[]  SumI2OutMin=[]  SumI2OutMax=[]  SumI3OutMin=[]  SumI3OutMax=[]  SumDOutMin=[]  SumDOutMax=[]  SaturationOutMin=[]  SaturationOutMax=[]  IntegratorContinuousStateAttributes=''  IntegratorStateMustResolveToSignalObject=off  IntegratorRTWStateStorageClass=Auto  FilterContinuousStateAttributes=''  FilterStateMustResolveToSignalObject=off  FilterRTWStateStorageClass=Auto  DifferentiatorICPrevScaledInput=0  DifferentiatorOutMin=[]  DifferentiatorOutMax=[]  FilterDiffOutCoefMin=[]  FilterDiffOutCoefMax=[]  SumDenOutMin=[]  SumDenOutMax=[]  SumNumOutMin=[]  SumNumOutMax=[]  ReciprocalOutMin=[]  ReciprocalOutMax=[]  DivideOutMin=[]  DivideOutMax=[]  TunerSelectOption=Transfer Function Based (PID Tuner App)
  Saturation : Saturate  UpperLimit=9.788  LowerLimit=-9.788
  Subsystem : Subsystem
  Subsystem2 : Subsystem
  Sum : Sum  Inputs=|+-
  Sum1 : Sum  Inputs=|+-
  Terminator2 : Terminator
  Terminator3 : Terminator
  Unit Delay1 : UnitDelay  SampleTime=-1
  gyro : Subsystem
  rate_d : Demux  Outputs=3
  舵机偏角输入eso : Subsystem
  ActuatorsBus : Outport  OutDataTypeStr=Bus: ActuatorsBus
  wires:
  PID Controller/1 -> Mux/3
  Bus Selector/3 -> Sum/1  "<yaw_cmd>"
  Demux/3 -> Sum/2
  PID Controller (2DOF)7/1 -> Saturation/1
  Bus Selector/2 -> PID Controller (2DOF)1/1  "<pitch_cmd>"
  Bus Selector1/2 -> Demux1/1, 舵机偏角输入eso/6(<pqr>)  "<Omega_body>"
  Sum/1 -> MATLAB Function1/1(u)
  PID Controller (2DOF)/1 -> Mux/1
  Demux3/2 -> Terminator2/1
  Demux/2 -> PID Controller (2DOF)1/2, Mux/5, Subsystem/1(In1)
  Demux1/2 -> gyro/4(q), PID Controller (2DOF)5/2
  rate_d/3 -> PID Controller (2DOF)6/1
  PID Controller (2DOF)1/1 -> Mux/2
  Demux1/3 -> PID Controller (2DOF)6/2
  MATLAB Function1/1(y) -> PID Controller/1
  Demux3/1 -> Terminator3/1
  rate_d/2 -> PID Controller (2DOF)5/1
  Bus Selector/4 -> PID Controller (2DOF)7/1  "<throttle_cmd>"
  rate_d/1 -> Sum1/1
  Mux/1 -> MATLAB Function/1(u)
  Command/1 -> Bus Selector/1
  Bus Creator/1 -> ActuatorsBus/1  "ActuatorsBus"
  Constant1/1 -> N-Sample Switch/1
  Subsystem/1(speed) -> N-Sample Switch/2  "speed"
  N-Sample Switch/1 -> gyro/6(speed), Bus Creator/5  "speed"
  Demux3/3 -> PID Controller (2DOF)7/2  "h"
  MATLAB Function/1(y) -> rate_d/1
  States/1 -> Unit Delay1/1
  Unit Delay1/1 -> Bus Selector1/1
  Add/1 -> Subsystem/3(In3)  "a_t"
  Constant/1 -> Add/1
  Sum1/1 -> Discrete PID Controller/1
  Bus Selector/1 -> PID Controller (2DOF)/1  "<roll_cmd>"
  Saturation/1 -> Add/2
  Demux/1 -> PID Controller (2DOF)/2, Subsystem/2(In2), Mux/4
  Demux1/1 -> gyro/2(p), Sum1/2
  Subsystem2/5(c1) -> Bus Creator/1
  Subsystem2/7(c3) -> Bus Creator/3
  Subsystem2/6(c2) -> Bus Creator/2
  Bus Selector1/3 -> Demux3/1  "<X_ned>"
  Subsystem2/8(c4) -> Bus Creator/4
  Bus Selector1/1 -> Demux/1, 舵机偏角输入eso/5(<Euler>)  "<<Euler>>"
  Discrete PID Controller/1 -> gyro/1(u_p)
  PID Controller (2DOF)5/1 -> gyro/3(u_q)
  PID Controller (2DOF)6/1 -> gyro/5(u_r)
  Demux2/1 -> Subsystem2/4(u_4)
  Demux2/2 -> Subsystem2/5(u_5)
  Demux2/3 -> Subsystem2/6(u_6)
  Subsystem2/1(c5) -> 舵机偏角输入eso/1(c1)
  Subsystem2/2(c6) -> 舵机偏角输入eso/2(c2)
  Subsystem2/3(c7) -> 舵机偏角输入eso/3(c3)
  Subsystem2/4(c8) -> 舵机偏角输入eso/4(c4)
  gyro/1(u_1) -> Subsystem2/1(u_1)
  gyro/2(u_2) -> Subsystem2/2(u_2)
  gyro/3(u_3) -> Subsystem2/3(u_3)
  舵机偏角输入eso/8(反馈) -> Demux2/1

== system flightSimulation/Visualization/Airspeed Indicator ==

== system flightSimulation/Visualization/Altimeter ==

== system flightSimulation/Visualization/Artificial Horizon ==

== system flightSimulation/Visualization/Climb Rate Indicator ==

== system flightSimulation/Visualization/Extract Flight Instruments ==
  States : Inport
  Altitude [ft] : aerolibconvert2/Length Conversion  IU=m  OU=ft
  Altitude [m] : Selector  InputPortWidth=3  IndexOptions=Index vector (dialog)  Indices=[3]  OutputSizes=1
  Bus Selector : BusSelector  OutputSignals=LLA,Euler,V_ned,V_body
  Demux : Demux  Outputs=3
  Display{,1..4} (5 alike) : Display
  Euler [deg] : aerolibconvert2/Angle Conversion  IU=rad  OU=deg
  Gain : Gain  Gain=-1/1000
  Math Function : Math  Operator=square  SaturateOnIntegerOverflow=on
  Mux : Mux  Inputs=2
  Sqrt : Sqrt  SaturateOnIntegerOverflow=on
  Sum of Elements : Sum  Inputs=+
  V : aerolibconvert2/Velocity Conversion  IU=m/s  OU=kts
  Vd [ft/min] : aerolibconvert2/Velocity Conversion  IU=m/s  OU=ft/min
  Vd [m/s] : Selector  InputPortWidth=3  IndexOptions=Index vector (dialog)  Indices=[3]  OutputSizes=1
  wires:
  Bus Selector/1 -> Altitude [m]/1  "<LLA>"
  Altitude [m]/1 -> Altitude [ft]/1
  States/1 -> Bus Selector/1
  Altitude [ft]/1 -> Display/1
  Bus Selector/2 -> Euler [deg]/1  "<Euler>"
  Euler [deg]/1 -> Demux/1
  Demux/1 -> Mux/1
  Demux/2 -> Mux/2
  Mux/1 -> Display1/1
  Demux/3 -> Display2/1
  Bus Selector/3 -> Vd [m/s]/1  "<V_ned>"
  Vd [m/s]/1 -> Vd [ft/min]/1
  Vd [ft/min]/1 -> Gain/1
  Gain/1 -> Display3/1
  Math Function/1 -> Sum of Elements/1
  Sum of Elements/1 -> Sqrt/1
  Bus Selector/4 -> Math Function/1  "<V_body>"
  Sqrt/1 -> V/1
  V/1 -> Display4/1

== system flightSimulation/Visualization/Heading Indicator ==

== system flightSimulation/Visualization/Visualization ==
  note: VSS_VISUALIZATION = 0 will select scopes as means to visualie variables/states
      | VSS_VISUALIZATION = 1 will send select states in a variable to the workspace
      | VSS_VISUALIZATION = 2 will use FlightGear as visualization
      | VSS_VISUALIZATION = 3 will use a Simulink 3D interface
  States : Inport  OutDataTypeStr=Bus: StatesBus
  Commands : Inport  Port=2  OutDataTypeStr=Bus: CommandBus
  FlightGear : Subsystem  VariantControl=VSS_VISUALIZATION_FLIGHTGEAR
      mask init:
      | visualizationFlightGearVars;
  Scopes : Subsystem  VariantControl=VSS_VISUALIZATION_SCOPES
  Simulink 3D : Subsystem  VariantControl=VSS_VISUALIZATION_SL3D
      mask init:
      | visualizationFlightGearVars;
  Workspace : Subsystem  VariantControl=VSS_VISUALIZATION_WORKSPACE

== system flightSimulation/senser/noise ==
  In1 : Inport
  Analog Filter Design : dsparch4/Analog Filter Design  method=Butterworth  filttype=Lowpass  N=2  Wlo=30*2*pi  Whi=80  Rp=2  Rs=40
  Analog Filter Design1 : dsparch4/Analog Filter Design  method=Butterworth  filttype=Lowpass  N=2  Wlo=30*2*pi  Whi=80  Rp=2  Rs=40
  Analog Filter Design2 : dsparch4/Analog Filter Design  method=Butterworth  filttype=Lowpass  N=2  Wlo=30*2*pi  Whi=80  Rp=2  Rs=40
  Colored Noise : dspsrcs4/Colored Noise  Color=custom  InverseFrequencyPower=1.55  NumChannels=1  OutputDataType=double  SamplesPerFrame=1  SampleTime=0.005  RandomStream=mt19937ar with seed  Seed=randperm(100000,1)  SimulateUsing=Interpreted execution
      settings: SourceProductName=DSP System Toolbox  SourceProductBaseCode=DS
  Colored Noise1 : dspsrcs4/Colored Noise  Color=custom  InverseFrequencyPower=1.55  NumChannels=1  OutputDataType=double  SamplesPerFrame=1  SampleTime=0.005  RandomStream=mt19937ar with seed  Seed=randperm(100000,1)  SimulateUsing=Interpreted execution
      settings: SourceProductName=DSP System Toolbox  SourceProductBaseCode=DS
  Colored Noise2 : dspsrcs4/Colored Noise  Color=custom  InverseFrequencyPower=1  NumChannels=1  OutputDataType=double  SamplesPerFrame=1  SampleTime=0.005  RandomStream=mt19937ar with seed  Seed=randperm(100000,1)  SimulateUsing=Interpreted execution
      settings: SourceProductName=DSP System Toolbox  SourceProductBaseCode=DS
  Demux : Demux  Outputs=3
  Gain : Gain  Gain=0.003
  Gain1 : Gain  Gain=0.003
  Gain2 : Gain  Gain=0.0025
  Mux : Mux  Inputs=3
  Mux1 : Mux  Inputs=2
  Mux2 : Mux  Inputs=2
  Mux3 : Mux  Inputs=2
  Random Number : RandomNumber  Variance=1.8365e-4  Seed=randperm(100000,1)
  Random Number1 : RandomNumber  Variance=1e-4  Seed=randperm(100000,1)
  Random Number2 : RandomNumber  Variance=1.4679e-6  Seed=randperm(100000,1)
  Scope3 : Scope  NumInputPorts=3
  Sum1 : Sum  Inputs=|++
  Sum3 : Sum  Inputs=|++
  Sum4 : Sum  Inputs=|++
  Out1 : Outport
  wires:
  In1/1 -> Demux/1
  Mux/1 -> Out1/1
  Demux/1 -> Sum1/2
  Demux/2 -> Sum3/2
  Demux/3 -> Sum4/2
  Sum1/1 -> Mux1/1, Analog Filter Design/1
  Sum3/1 -> Mux2/1, Analog Filter Design1/1
  Sum4/1 -> Mux3/1, Analog Filter Design2/1
  Mux3/1 -> Scope3/3
  Mux2/1 -> Scope3/2
  Mux1/1 -> Scope3/1
  Colored Noise/1 -> Gain/1
  Colored Noise1/1 -> Gain1/1
  Gain1/1 -> Sum3/1
  Colored Noise2/1 -> Gain2/1
  Gain2/1 -> Sum4/1
  Analog Filter Design/1 -> Mux/1, Mux1/2
  Analog Filter Design1/1 -> Mux/2, Mux2/2
  Analog Filter Design2/1 -> Mux/3, Mux3/2
  Gain/1 -> Sum1/1

== system flightSimulation/Command/Signal Builder/Signal Builder ==
  Demux : Demux  Tag=STV Demux
  FromWs : FromWorkspace  Tag=STV FromWs  VariableName=tuvar  SampleTime=0
      SigBuilderData=|
      | common.afterFinalStr = 'Extrapolate'
      | common.sampleTime = 0
      | dataSet.timeRange = [0 80]
      | dataSet.name = 'Group 1'
      | sbobj.Groups.Name = 'Group 1'
      | sbobj.Groups.Signals(1).Name = 'roll_cmd'
      | sbobj.Groups.Signals(1).XData = [0 0.3 11 11 21.6 21.6 80]
      | sbobj.Groups.Signals(1).YData = [0 0 0 0.349065850399 0.349065850399 0 0]
      | sbobj.Groups.Signals(2).Name = 'picth_cmd'
      | sbobj.Groups.Signals(2).XData = [0 11 11 26.3 26.3 80]
      | sbobj.Groups.Signals(2).YData = [0 0 0.349065850399 0.349065850399 0 0]
      | sbobj.Groups.Signals(3).Name = 'yaw_cmd'
      | sbobj.Groups.Signals(3).XData = [0 21.4 21.4 24.1 24.1 80]
      | sbobj.Groups.Signals(3).YData = [0 0 1 1 0 0]
      | sbobj.Groups.Signals(4).Name = 'throttle_cmd'
      | sbobj.Groups.Signals(4).XData = [0 80]
      | sbobj.Groups.Signals(4).YData = [0 0]
      | sbobj.Groups.TimeRange = [0 80]
  roll_cmd : Outport  Tag=STV Outport
  picth_cmd : Outport  Tag=STV Outport  Port=2
  yaw_cmd : Outport  Tag=STV Outport  Port=3
  throttle_cmd : Outport  Tag=STV Outport  Port=4
  wires:
  Demux/1 -> roll_cmd/1
  FromWs/1 -> Demux/1
  Demux/2 -> picth_cmd/1
  Demux/3 -> yaw_cmd/1
  Demux/4 -> throttle_cmd/1

== system flightSimulation/Command/Subsystem/Signal Builder ==
  Demux : Demux  Tag=STV Demux
  FromWs : FromWorkspace  Tag=STV FromWs  VariableName=tuvar  SampleTime=0
      SigBuilderData=|
      | common.afterFinalStr = 'Extrapolate'
      | common.sampleTime = 0
      | dataSet.timeRange = [0 80]
      | dataSet.name = 'Group 1'
      | sbobj.Groups.Name = 'Group 1'
      | sbobj.Groups.Signals(1).Name = 'roll_cmd'
      | sbobj.Groups.Signals(1).XData = [0 0.3 21.9 21.9 27.4 27.4 80]
      | sbobj.Groups.Signals(1).YData = [0 0 0 0.011 0.011 0 0]
      | sbobj.Groups.Signals(2).Name = 'picth_cmd'
      | sbobj.Groups.Signals(2).XData = [0 15.5 15.5 20.3 20.3 80]
      | sbobj.Groups.Signals(2).YData = [0 0 0.349065850399 0.349065850399 0 0]
      | sbobj.Groups.Signals(3).Name = 'yaw_cmd'
      | sbobj.Groups.Signals(3).XData = [0 14 14 17.3 17.3 80]
      | sbobj.Groups.Signals(3).YData = [0 0 1 1 0 0]
      | sbobj.Groups.Signals(4).Name = 'throttle_cmd'
      | sbobj.Groups.Signals(4).XData = [0 80]
      | sbobj.Groups.Signals(4).YData = [0 0]
      | sbobj.Groups.TimeRange = [0 80]
  roll_cmd : Outport  Tag=STV Outport
  picth_cmd : Outport  Tag=STV Outport  Port=2
  yaw_cmd : Outport  Tag=STV Outport  Port=3
  throttle_cmd : Outport  Tag=STV Outport  Port=4
  wires:
  Demux/1 -> roll_cmd/1
  FromWs/1 -> Demux/1
  Demux/2 -> picth_cmd/1
  Demux/3 -> yaw_cmd/1
  Demux/4 -> throttle_cmd/1

== system flightSimulation/Command/Subsystem/Signal Builder1 ==
  Demux : Demux  Tag=STV Demux
  FromWs : FromWorkspace  Tag=STV FromWs  VariableName=tuvar  SampleTime=0
      SigBuilderData=|
      | common.afterFinalStr = 'Extrapolate'
      | common.sampleTime = 0
      | dataSet.timeRange = [0 20]
      | dataSet.name = 'Group 1'
      | sbobj.Groups.Name = 'Group 1'
      | sbobj.Groups.Signals(1).Name = 'roll_cmd'
      | sbobj.Groups.Signals(1).XData = [0 1 1 3 3 6 6 7 7 10 10 11 11 12 12 13 13 15 15 20]
      | sbobj.Groups.Signals(1).YData = [0.03 0.03 -0.025 -0.025 0.02 0.02 -0.02 -0.02 0.018 0.018 -0.02 -0.02 0.016 0.016 -0.02 -0.02 0.01 0.01 -0.02 -0.02]
      | sbobj.Groups.Signals(2).Name = 'pitch_cmd'
      | sbobj.Groups.Signals(2).XData = [0 0.5 0.5 1 1 2.5 2.5 3 3 4.5 4.5 7.5 7.5 8 8 8.5 8.5 9 9 9.5 9.5 12 12 12.5 12.5 13 13 13.5 13.5 14.5 14.5 16 16 17.5 17.5 20]
      | sbobj.Groups.Signals(2).YData = [0.026 0.026 -0.008 -0.008 0.016 0.016 -0.008 -0.008 0.018 0.018 -0.01 -0.01 0.02 0.02 -0.012 -0.012 0.012 0.012 -0.008 -0.008 0.018 0.018 -0.01 -0.01 0.023 0.023 -0.008 -0.008 0.014 0.014 -0.007 -0.007 0.015 0.015 -0.014 -0.014]
      | sbobj.Groups.Signals(3).Name = 'yaw_cmd'
      | sbobj.Groups.Signals(3).XData = [0 1 2 3 4 5 6 7 8 9 10 11 12 13 14 15 16 17 18 19 20]
      | sbobj.Groups.Signals(3).YData = [-0.0171604702497 0.0125759574715 -0.0118415584332 0.00281644961979 0.00914349459385 0.00482747657739 0.00373550607694 -0.0086447642033 -0.000550505225013 0.00930401081905 -0.00763580794482 -0.0123569780611 -0.00698666763789 0.0085444103418 -0.00274565612232 0.00222871093046 -0.0174483453587 -0.00772631263063 -0.00699480510364 -0.0126593037272 0.0117396852628]
      | sbobj.Groups.Signals(4).Name = 'throttle_cmd'
      | sbobj.Groups.Signals(4).XData = [0 20]
      | sbobj.Groups.Signals(4).YData = [0 0]
      | sbobj.Groups.TimeRange = [0 20]
  roll_cmd : Outport  Tag=STV Outport
  pitch_cmd : Outport  Tag=STV Outport  Port=2
  yaw_cmd : Outport  Tag=STV Outport  Port=3
  throttle_cmd : Outport  Tag=STV Outport  Port=4
  wires:
  FromWs/1 -> Demux/1
  Demux/1 -> roll_cmd/1
  Demux/2 -> pitch_cmd/1
  Demux/3 -> yaw_cmd/1
  Demux/4 -> throttle_cmd/1

== system flightSimulation/Nonlinear/Plant/Bus setup ==
  LLA : Inport  PortDimensions=3
  V_ned : Inport  Port=2  PortDimensions=3
  X_ned : Inport  Port=3  PortDimensions=3
  Euler : Inport  Port=4  PortDimensions=3
  DCM_be : Inport  Port=5  PortDimensions=[3 3]
  V_b : Inport  Port=6  PortDimensions=3
  Omega_b : Inport  Port=7  PortDimensions=3
  dOmega_b : Inport  Port=8  PortDimensions=3
  Accel_b : Inport  Port=9  PortDimensions=3
  Bus Creator5 : BusCreator  Inputs=9  OutDataTypeStr=Bus: StatesBus  NonVirtualBus=on
  States : Outport
  wires:
  Bus Creator5/1 -> States/1
  V_b/1 -> Bus Creator5/1  "V_body"
  Omega_b/1 -> Bus Creator5/2  "Omega_body"
  Euler/1 -> Bus Creator5/3  "Euler"
  X_ned/1 -> Bus Creator5/7  "X_ned"
  Accel_b/1 -> Bus Creator5/4  "Accel_body"
  LLA/1 -> Bus Creator5/8  "LLA"
  dOmega_b/1 -> Bus Creator5/5  "dOmega_body"
  DCM_be/1 -> Bus Creator5/9  "DCM_be"
  V_ned/1 -> Bus Creator5/6  "V_ned"

== system flightSimulation/Nonlinear/Plant/Position on Earth ==
  Xe : Inport
  Flat Earth to LLA : aerolibtransform2/Flat Earth to LLA  units=Metric (MKS)  ptype=Earth (WGS84)  F=1/298.257223563  R=6378137  LL0=initPosLLA(1:2)  psi=Vehicle.Nonlinear.Nonlinear.PositionOnEarth.FlatEarthToLLA.xAxis
  Mux : Mux  Inputs=2
  href : Constant  Value=Vehicle.Nonlinear.Nonlinear.PositionOnEarth.href
  LLA : Outport
  wires:
  Mux/1 -> LLA/1
  Xe/1 -> Flat Earth to LLA/1
  Flat Earth to LLA/1 -> Mux/1
  Flat Earth to LLA/2 -> Mux/2
  href/1 -> Flat Earth to LLA/2

== system flightSimulation/Nonlinear/Plant/Subsystem ==
  ActuatorsBus : Inport
  EnvironmentBus : Inport  Port=2
  Bus Selector : BusSelector  OutputSignals=speed,c1,c2,c3,c4
  Bus Selector1 : BusSelector  OutputSignals=StatesBus.V_body,Wind_ned,Gravity_ned,StatesBus.DCM_be
  Demux : Demux  Outputs=3
  Demux1 : Demux  Outputs=3
  Mux1 : Mux  Inputs=11
  S-Function : S-Function  FunctionName=s_Force  SFunctionDeploymentMode=off  EnableBusSupport=off
  Subsystem1 : Subsystem
  Out1 : Outport
  wires:
  ActuatorsBus/1 -> Bus Selector/1
  Demux/1 -> Mux1/6
  Demux/2 -> Mux1/7
  Mux1/1 -> S-Function/1
  Bus Selector/3 -> Mux1/3  "<c2>"
  Bus Selector1/4 -> Subsystem1/3(Rn2b)  "<DCM_be>"
  Demux1/1 -> Mux1/9
  Demux1/3 -> Mux1/11
  Demux1/2 -> Mux1/10
  Bus Selector/5 -> Mux1/5  "<c4>"
  EnvironmentBus/1 -> Bus Selector1/1
  Bus Selector/1 -> Mux1/1  "<speed>"
  Bus Selector/4 -> Mux1/4  "<c3>"
  Demux/3 -> Mux1/8
  Bus Selector1/2 -> Demux1/1  "<Wind_ned>"
  Bus Selector1/1 -> Demux/1  "<V_body>"
  Bus Selector/2 -> Mux1/2  "<c1>"
  Bus Selector1/3 -> Subsystem1/2(g_ned)  "<Gravity_ned>"
  Subsystem1/1(F_b) -> Out1/1
  S-Function/1 -> Subsystem1/1(F)

== system flightSimulation/Nonlinear/Plant/Subsystem1 ==
  In1 : Inport  OutDataTypeStr=Bus: ActuatorsBus
  In2 : Inport  Port=2  OutDataTypeStr=Bus: EnvironmentBus
  Bus Selector1 : BusSelector  OutputSignals=StatesBus.V_body,Wind_ned,StatesBus.Omega_body,StatesBus.Euler
  Bus Selector2 : BusSelector  OutputSignals=c1,c2,c3,c4,speed
  Demux : Demux  Outputs=3
  Demux1 : Demux  Outputs=3
  Demux2 : Demux  Outputs=3
  Demux3 : Demux  Outputs=6
  M : S-Function  FunctionName=s_Torque  SFunctionDeploymentMode=off  EnableBusSupport=off
  Mux : Mux  Inputs=3
  Mux2 : Mux  Inputs=17
  To Workspace : ToWorkspace  VariableName=turbulent  SaveFormat=Timeseries  SampleTime=-1
  扰动 : Mux  Inputs=3
  Out1 : Outport
  wires:
  Demux1/3 -> Mux2/11
  Mux2/1 -> M/1
  Demux1/2 -> Mux2/10
  Demux/3 -> Mux2/8
  Bus Selector2/3 -> Mux2/3  "<c3>"
  Demux/1 -> Mux2/6
  Bus Selector2/5 -> Mux2/5  "<speed>"
  M/1 -> Demux3/1
  Demux1/1 -> Mux2/9
  Bus Selector2/4 -> Mux2/4  "<c4>"
  Demux/2 -> Mux2/7
  Demux2/2 -> Mux2/13
  In1/1 -> Bus Selector2/1  "ActuatorsBus"
  In2/1 -> Bus Selector1/1  "EnvironmentBus"
  Bus Selector2/1 -> Mux2/1  "<c1>"
  Bus Selector2/2 -> Mux2/2  "<c2>"
  Bus Selector1/1 -> Demux/1  "<V_body>"
  Bus Selector1/2 -> Demux1/1  "<Wind_ned>"
  Bus Selector1/3 -> Demux2/1  "<Omega_body>"
  Demux2/1 -> Mux2/12
  Demux3/6 -> 扰动/3  "偏航_扰动"
  Demux3/5 -> 扰动/2  "俯仰_扰动"
  Demux3/4 -> 扰动/1  "滚转_扰动"
  Demux3/1 -> Mux/1
  Demux3/2 -> Mux/2
  Demux3/3 -> Mux/3
  Mux/1 -> Out1/1
  扰动/1 -> To Workspace/1  "真实扰动"
  Demux2/3 -> Mux2/14

== system flightSimulation/Subsystem/ADRC_allocator/Subsystem ==
  q : Inport
  p : Inport  Port=2
  In3 : Inport  Port=3
  Divide : Product  Inputs=*/
  Gain : Gain  Gain=-1225^2/9.788
  Product : Product
  Saturation1 : Saturate  UpperLimit=1  LowerLimit=0.5
  Sqrt : Sqrt  SaturateOnIntegerOverflow=on
  Trigonometric Function : Trigonometry  Operator=cos
  Trigonometric Function1 : Trigonometry  Operator=cos
  speed : Outport
  wires:
  Saturation1/1 -> Divide/2
  Trigonometric Function/1 -> Product/1
  In3/1 -> Divide/1
  Trigonometric Function1/1 -> Product/2
  p/1 -> Trigonometric Function/1
  Product/1 -> Saturation1/1
  q/1 -> Trigonometric Function1/1
  Divide/1 -> Gain/1
  Gain/1 -> Sqrt/1
  Sqrt/1 -> speed/1

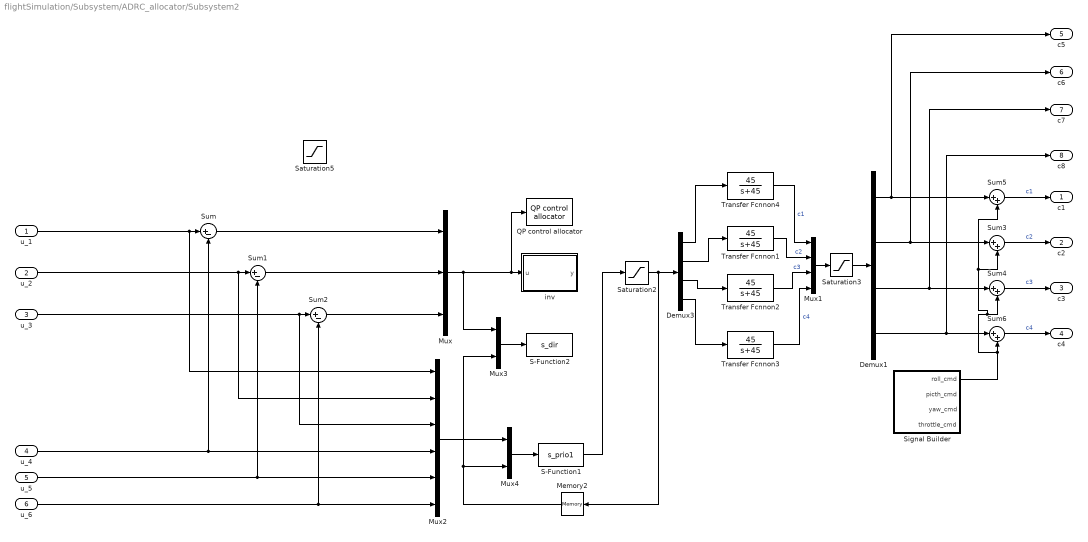
== system flightSimulation/Subsystem/ADRC_allocator/Subsystem2 ==
  u_1 : Inport
  u_2 : Inport  Port=2
  u_3 : Inport  Port=3
  u_4 : Inport  Port=4
  u_5 : Inport  Port=5
  u_6 : Inport  Port=6
  Demux1 : Demux
  Demux3 : Demux
  Memory2 : Memory  InitialCondition=[0;0;0;0]  InheritSampleTime=on  LinearizeAsDelay=on
  Mux : Mux  Inputs=3
  Mux1 : Mux
  Mux2 : Mux  Inputs=6
  Mux3 : Mux  Inputs=2
  Mux4 : Mux  Inputs=2
  QP control allocator : qcatlib/QP control allocator  B=B  plim=[umin umax]  rlim=[]  T=0.01  Wv=eye(3)  Wu=eye(4)  ud=zeros(4,1)  alg=WLS  imax=100  gam=1e6  tol=1e-4
      settings: SourceProductName=QP Control Allocation Toolbox
  S-Function1 : S-Function  FunctionName=s_prio1  SFunctionDeploymentMode=off  EnableBusSupport=off
  S-Function2 : S-Function  FunctionName=s_dir  SFunctionDeploymentMode=off  EnableBusSupport=off
  Saturation2 : Saturate  UpperLimit=umax  LowerLimit=umin
  Saturation3 : Saturate  UpperLimit=umax  LowerLimit=umin
  Saturation5 : Saturate  UpperLimit=p_limits*pi/180  LowerLimit=-p_limits*pi/180
  Signal Builder : Subsystem  Tag=STV Subsys  LoadFcn=sigbuilder_block('load');  StartFcn=sigbuilder_block('start');  StopFcn=sigbuilder_block('stop');  ClipboardFcn=sigbuilder_block('clipboard');  mask(Sigbuilder block){tuvar=[0:10]}
      mask help: Simulink:masks:SigbuilderBlock_MD
      mask init:
      | if ~strcmp(get_param(bdroot(gcbh),'SimulationStatus'),'stopped') tuvar = sigbuilder_block('maskInit'); end
      settings: CopyFcn=sigbuilder_block('copy');  DeleteFcn=sigbuilder_block('delete');  ModelCloseFcn=sigbuilder_block('modelClose');  PreSaveFcn=sigbuilder_block('preSave');  PauseFcn=sigbuilder_block('pause');  ContinueFcn=sigbuilder_block('continue');  NameChangeFcn=sigbuilder_block('namechange');  OpenFcn=sigbuilder_block('open',[75 129 943.5 382.5 ]);  CloseFcn=sigbuilder_block('close');
      mask Display: plot(0, 0, 100, 100,[2, 2, 32, 32, 2], [68, 8, 8, 68, 68],[32, 2], [38, 38], [32, 19, 2],[53, 60, 44], [32, 17, 17, 2],[16, 16, 31, 31]);txt = getActiveGroup(gcbh);text(2, 100, txt,'verticalAlignment', 'top');
  Sum : Sum  Inputs=|+-
  Sum1 : Sum  Inputs=|+-
  Sum2 : Sum  Inputs=|+-
  Sum{3..6} (4 alike) : Sum  Inputs=|++
  Transfer Fcnnon{1..4} (4 alike) : TransferFcn  Numerator=45  Denominator=[1 45]
  inv : MATLAB Function  TreatAsAtomicUnit=on
  c1 : Outport
  c2 : Outport  Port=2
  c3 : Outport  Port=3
  c4 : Outport  Port=4
  c5 : Outport  Port=5
  c6 : Outport  Port=6
  c7 : Outport  Port=7
  c8 : Outport  Port=8
  wires:
  u_3/1 -> Mux2/3, Sum2/1
  u_1/1 -> Mux2/1, Sum/1
  u_2/1 -> Mux2/2, Sum1/1
  Sum2/1 -> Mux/3
  Sum/1 -> Mux/1
  Sum1/1 -> Mux/2
  u_4/1 -> Mux2/4, Sum/2
  u_5/1 -> Mux2/5, Sum1/2
  u_6/1 -> Mux2/6, Sum2/2
  Sum5/1 -> c1/1  "c1"
  Sum3/1 -> c2/1  "c2"
  Sum4/1 -> c3/1  "c3"
  Sum6/1 -> c4/1  "c4"
  Demux3/1 -> Transfer Fcnnon4/1
  Demux3/2 -> Transfer Fcnnon1/1
  Demux3/3 -> Transfer Fcnnon2/1
  Demux3/4 -> Transfer Fcnnon3/1
  Mux/1 -> QP control allocator/1, inv/1(u), Mux3/1
  Mux2/1 -> Mux4/1
  Memory2/1 -> Mux3/2, Mux4/2
  Mux4/1 -> S-Function1/1
  Saturation3/1 -> Demux1/1
  Saturation2/1 -> Memory2/1, Demux3/1
  Mux1/1 -> Saturation3/1
  Transfer Fcnnon4/1 -> Mux1/1  "c1"
  Transfer Fcnnon1/1 -> Mux1/2  "c2"
  Transfer Fcnnon2/1 -> Mux1/3  "c3"
  Transfer Fcnnon3/1 -> Mux1/4  "c4"
  Demux1/1 -> Sum5/1, c5/1
  Demux1/2 -> Sum3/1, c6/1
  Demux1/3 -> Sum4/1, c7/1
  Demux1/4 -> Sum6/1, c8/1
  Mux3/1 -> S-Function2/1
  Signal Builder/1(roll_cmd) -> Sum5/2, Sum3/2, Sum4/2, Sum6/2
  S-Function1/1 -> Saturation2/1
